simulink subsystem "Visualizer"  (R2023b)
settings: Solver=VariableStepAuto  StartTime=0.0  StopTime=10.0  RelTol=1e-3
libraries: robotcorelib x1, uavutilslib x1
settings Model: Creator=luke  LastModifiedBy=luke

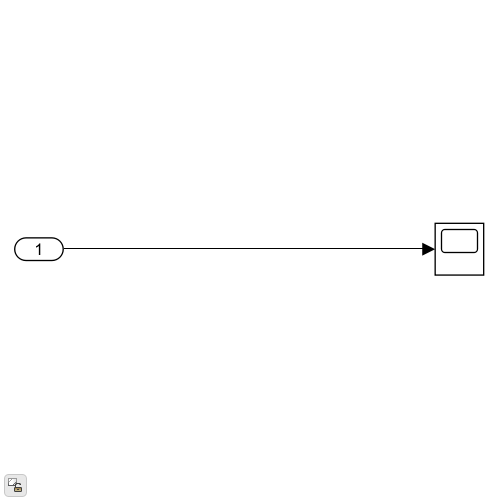
[thumbnail: Simulink's stored preview of the top-level diagram]
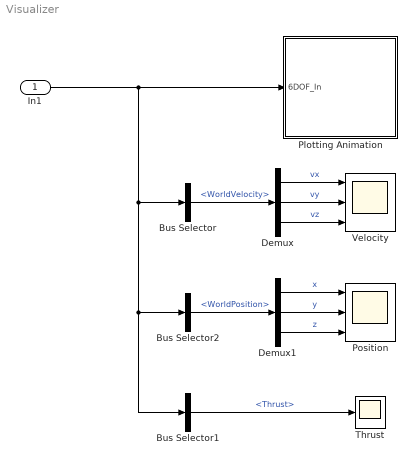
== system Visualizer ==
  In1 : Inport  OutDataTypeStr=Bus: StateBus
  Bus Selector : BusSelector  OutputSignals=WorldVelocity
  Bus Selector1 : BusSelector  OutputSignals=Thrust
  Bus Selector2 : BusSelector  OutputSignals=WorldPosition
  Demux : Demux  Outputs=3
  Demux1 : Demux  Outputs=3
  Plotting Animation : Subsystem  Variant=on
      mask Display: disp('Plotting Animation');
  Position : Scope  NumInputPorts=3
  Thrust : Scope
  Velocity : Scope  NumInputPorts=3
  wires:
  Bus Selector1/1 -> Thrust/1  "<Thrust>"
  Bus Selector/1 -> Demux/1  "<WorldVelocity>"
  Demux/3 -> Velocity/3  "vz"
  Demux/2 -> Velocity/2  "vy"
  Demux/1 -> Velocity/1  "vx"
  Demux1/2 -> Position/2  "y"
  Bus Selector2/1 -> Demux1/1  "<WorldPosition>"
  Demux1/1 -> Position/1  "x"
  Demux1/3 -> Position/3  "z"
  In1/1 -> Plotting Animation/1(6DOF_In), Bus Selector1/1, Bus Selector2/1, Bus Selector/1

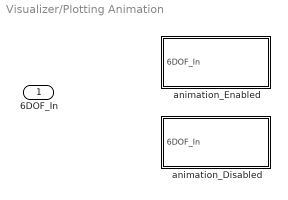
== system Visualizer/Plotting Animation ==
  6DOF_In : Inport  OutDataTypeStr=Bus: StateBus
  animation_Disabled : Subsystem  VariantControl=userInputs.Visualization.animation == 0
      mask Display: disp('Animation Disabled');
  animation_Enabled : Subsystem  VariantControl=userInputs.Visualization.animation == 1
      mask Display: disp('Animation Enabled');

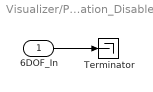
== system Visualizer/Plotting Animation/animation_Disabled ==
  6DOF_In : Inport
  Terminator : Terminator
  wires:
  6DOF_In/1 -> Terminator/1

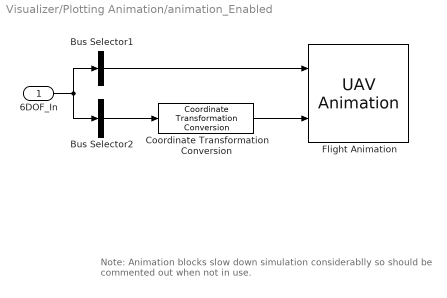
== system Visualizer/Plotting Animation/animation_Enabled ==
  note: Note: Animation blocks slow down simulation considerablly so should be commented out when not in use.
  6DOF_In : Inport  OutDataTypeStr=Bus: StateBus
  Bus Selector1 : BusSelector  OutputSignals=WorldPosition  OutputAsBus=on
  Bus Selector2 : BusSelector  OutputSignals=EulerZYX  OutputAsBus=on
  Coordinate Transformation Conversion : robotcorelib/Coordinate Transformation Conversion  InputRepresentation=Euler Angles  InputEulerSequence=ZYX  ShowTrVecInputPort=on  OutputRepresentation=Quaternion  OutputEulerSequence=ZYX  ShowTrVecOutputPort=on  SimulateUsing=Interpreted execution
  Flight Animation : uavutilslib/UAV Animation  UAVType=FixedWing  UAVSize=0.1  InertialZDirection=Up  SampleTime=-1
  wires:
  Bus Selector2/1 -> Coordinate Transformation Conversion/1
  Bus Selector1/1 -> Flight Animation/1
  6DOF_In/1 -> Bus Selector2/1, Bus Selector1/1
  Coordinate Transformation Conversion/1 -> Flight Animation/2
